simulink model "full_motion_model"  (R2021b)
settings: Solver=VariableStepAuto  StartTime=0.0  StopTime=10.0  RelTol=1e-3
settings Model: Creator=den  LastModifiedBy=den

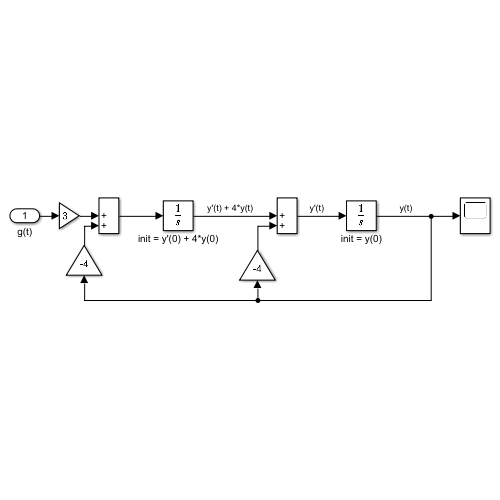
[thumbnail: Simulink's stored preview of the top-level diagram]
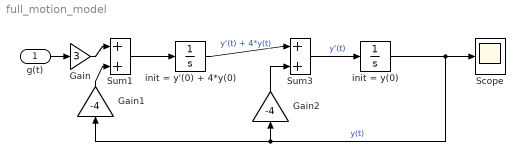
== system full_motion_model ==
  g(t) : Inport
  Gain : Gain  Gain=3
  Gain1 : Gain  Gain=-4
  Gain2 : Gain  Gain=-4
  Scope : Scope
  Sum1 : Sum  Inputs=|++
  Sum3 : Sum  Inputs=|++
  init = y'(0) + 4*y(0) : Integrator  InitialCondition=6
  init = y(0) : Integrator  InitialCondition=1
  wires:
  Gain1/1 -> Sum1/2
  Sum3/1 -> init = y(0)/1  "y'(t)"
  Gain2/1 -> Sum3/2
  init = y'(0) + 4*y(0)/1 -> Sum3/1  "y'(t) + 4*y(t)"
  init = y(0)/1 -> Gain1/1, Gain2/1, Scope/1  "y(t)"
  Sum1/1 -> init = y'(0) + 4*y(0)/1
  Gain/1 -> Sum1/1
  g(t)/1 -> Gain/1
